simulink model "DrogueVisualNavigation_2016b"  (R2016b)
settings: Solver=ode3  StartTime=0.0  StopTime=200  FixedStep=0.02  RelTol=1e-3  EnableMultiTasking=on
libraries: visionmorphops x2, visionsinks x1, vrlib x1
settings Model: Creator=daidai  LastModifiedBy=51078
settings DataIOCC: LimitDataPoints=on  SaveFormat=Array
settings OptimizationCC: LifeSpan=inf
settings DebuggingCC: UnderspecifiedInitializationDetection=Classic  MergeDetectMultiDrivingBlocksExec=none  SolverPrmCheckMsg=warning  StateNameClashWarn=warning  SFUnexpectedBacktrackingDiag=warning  SFNoUnconditionalDefaultTransitionDiag=warning  SFExecutionAtInitializationDiag=none
settings HardwareCC: ProdBitPerPointer=32  ProdBitPerSizeT=32  ProdBitPerPtrDiffT=32  ProdLargestAtomicFloat=None  ProdIntDivRoundTo=Undefined  ProdEndianess=Unspecified  ProdWordSize=32  ProdHWDeviceType=32-bit Generic
settings ModelReferenceCC: PropagateSignalLabelsOutOfModel=off
settings GRTTargetCC: TargetLangStandard=C89/C90 (ANSI)  GeneratePreprocessorConditionals=Disable all
settings ConfigComp: CovMetricSettings=dw  CovHtmlReporting=on  CovSaveCumulativeToWorkspaceVar=on  CovSaveSingleToWorkspaceVar=on  CovExternalEMLEnable=off

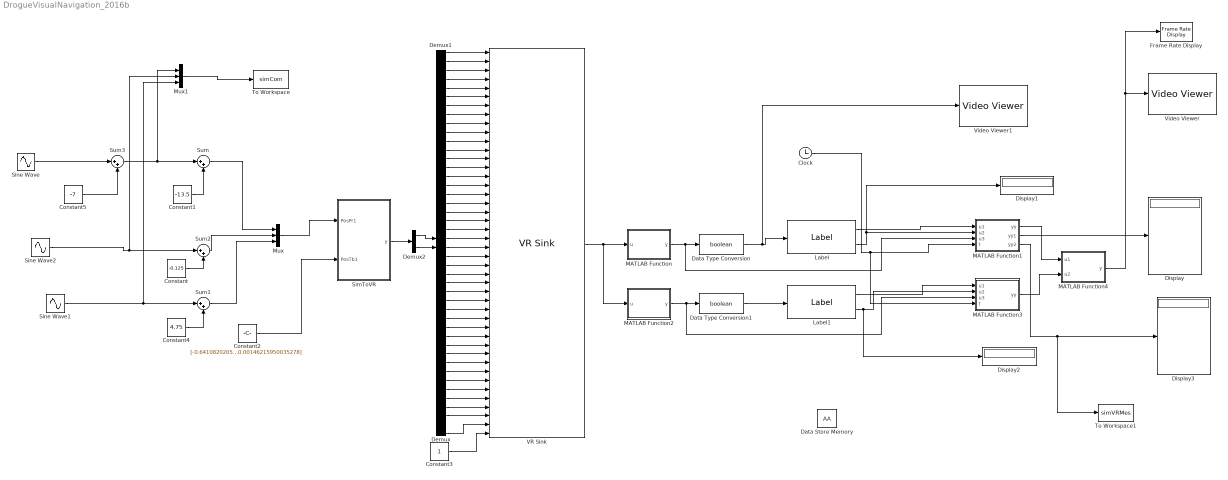
== system DrogueVisualNavigation_2016b ==
  Clock : Clock
  Constant : Constant  Value=-0.125
  Constant1 : Constant  Value=-13.5
  Constant2 : Constant  Value="[-0.641082020570737\t0.000198505356969816\t0.319485276494183\t-1.28393532402013\t-0.00160281843683540\t0.635386248124202\t-1.93123901470987\t-0.00236208899737502\t0.942069136345351\t-2.57908748233429\t-0.00371191186814384\t1.24759749734461\t-3.23222347389724\t-0.00458728864970563\t1.54165471735559\t-3.88606315497445\t-0.00765856664806413\t1.83412912153534\t-4.54441464916205\t-0.00690931267848755\t2.11631662501387\t-5.20488531429186\t-0.00757809487662455\t2.39350806000665\t-5.86949292725030\t-0.00976373475740374\t2.66062036256121\t-6.53599124911111\t-0.0104781906153184\t2.92298750019385\t-7.20684903813727\t-0.0123446852873486\t3.17399224417408\t-7.88023087161393\t-0.0124294906988970\t3.41815190003813\t-8.55684999137055\t-0.0142996532310569\t3.65318404182279\t-9.23697996759531\t-0.0159268140819394\t3.87785626126273\t-9.92032158813885\t-0.0164263298291676\t4.09256773863864\t-10.6066111675631\t-0.0169568013994899\t4.29766130307588\t-11.2962129353769\t-0.0151955417452362\t4.49131908937044\t-11.9886887378561\t-0.0139647208223945\t4.67443868542926\t-12.6842362038538\t-0.0162199773408155\t4.84551081864269\t-13.3827602154087\t-0.0151986230932412\t5.00400435326389\t0.462329282331198\t0.456745997324795\t0.442456410271379\t0.440673569146200\t0.423039498148698\t0.420617409284319\t0.404938855304994\t0.397362334614631\t0.382149787076285\t0.375020180752588\t0.358028304224740\t0.347844084701537\t0.334322083149496\t0.319050746042371\t0.304440174994498\t0.290395880255186\t0.273773209510574\t0.258523760775515\t0.241165090536005\t0.223119792668294\t-0.000309641113392978\t0.00280206863637395\t0.00117297371116799\t0.00208354420047296\t0.00134026645096743\t0.00469726065688700\t-0.00113807540912366\t0.00101258391155381\t0.00328860512426005\t0.00107195406323456\t0.00278224369822605\t0.000125939558930855\t0.00276397416973394\t0.00239242174777090\t0.000730989659109897\t0.000772955732654557\t-0.00255401872049031\t-0.00177741896870770\t0.00324240792373905\t-0.00146215950035278]"
  Constant3 : Constant
  Constant4 : Constant  Value=4.75
  Constant5 : Constant  Value=-7
  Data Store Memory : DataStoreMemory  DataStoreName=AA  InitialValue=[0 0 0]  ShowAdditionalParam=off  OutDataTypeStr=double
  Data Type Conversion : DataTypeConversion  OutDataTypeStr=boolean
  Data Type Conversion1 : DataTypeConversion  OutDataTypeStr=boolean
  Demux : Demux  Outputs=22
  Demux1 : Demux  Outputs=22
  Demux2 : Demux  Outputs=[88,66]
  Display{,1..3} (4 alike) : Display
  Frame Rate Display : visionsinks/Frame Rate Display  UpdateRate=10
  Label : visionmorphops/Label  conn=8  output=Label matrix and number of labels  outType=Automatic  lastLabel=maximum value of the output data type
  Label1 : visionmorphops/Label  conn=8  output=Label matrix and number of labels  outType=Automatic  lastLabel=maximum value of the output data type
  MATLAB Function : MATLAB Function  TreatAsAtomicUnit=on
  MATLAB Function1 : MATLAB Function  TreatAsAtomicUnit=on
  MATLAB Function2 : MATLAB Function  TreatAsAtomicUnit=on
  MATLAB Function3 : MATLAB Function  TreatAsAtomicUnit=on
  MATLAB Function4 : MATLAB Function  TreatAsAtomicUnit=on
  Mux : Mux  Inputs=3
  Mux1 : Mux  Inputs=3
  SimToVR : MATLAB Function  TreatAsAtomicUnit=on
  Sine Wave : Sin  Amplitude=7  SampleTime=0
  Sine Wave1 : Sin  Frequency=5  SampleTime=0
  Sine Wave2 : Sin  Frequency=3  SampleTime=0
  Sum{,1..3} (4 alike) : Sum  Inputs=|++
  To Workspace : ToWorkspace  VariableName=simCom  SampleTime=-1
  To Workspace1 : ToWorkspace  VariableName=simVRMes  SampleTime=-1
  VR Sink : vrlib/VR Sink  InstantiateOnLoad=on  SampleTime=-1  ViewEnable=on  RemoteChange=off  RemoteView=off  FieldsWritten=tube1.rotation.4.1.1.double#tube1.translation.3.1.1.double#tube2.rotation.4.1.1.double#tube2.translation.3.1.1.double#tube3.rotation.4.1.1.double#tube3.translation.3.1.1.double#tube4.rotation.4.1.1.double#tube4.translation.3.1.1.double#tube5.rotation.4.1.1.double#tube5.translation.3.1.1.double#tube6.rotation.4.1.1.double#tube6.translation.3.1.1.double#tube7.rotation.4.1.1.double#tube7.translation.3.1.1.double#tube8.rotation.4.1.1.double#tube8.translation.3.1.1.double#tube9.rotation.4.1.1.double#tube9.translation.3.1.1.double#tube10.rotation.4.1.1.double#tube10.translation.3.1.1.double#tube11.rotation.4.1.1.double#tube11.translation.3.1.1.double#tube12.rotation.4.1.1.double#tube12.translation.3.1.1.double#tube13.rotation.4.1.1.double#tube13.translation.3.1.1.double#tube14.rotation.4.1.1.double#tube14.translation.3.1.1.double#tube15.rotation.4.1.1.double#tube15.translation.3.1.1.double#tube16.rotation.4.1.1.double#tube16.translation.3.1.1.double#tube17.rotation.4.1.1.double#tube17.translation.3.1.1.double#tube18.rotation.4.1.1.double#tube18.translation.3.1.1.double#tube19.rotation.4.1.1.double#tube19.translation.3.1.1.double#tube20.rotation.4.1.1.double#tube20.translation.3.1.1.double#tube21.rotation.4.1.1.double#tube21.translation.3.1.1.double#ASDD.translation.3.1.1.double#ReceiverViewPoint.set_bind.1.1.1.logical  WorldFileName=AirRefuelingTubeSim.WRL  AutoView=off  VideoDimensions=[480 860]  AllowVariableSize=off  FigureProperties="{'Position', 'Name', 'Viewpoint', 'CameraBound', 'CameraDirection', 'CameraPosition', 'CameraUpVector', 'ZoomFactor', 'Antialiasing', 'Headlight', 'Lighting', 'NavPanel', 'Sound', 'StatusBar', 'Stereo3D', 'Stereo3DCameraOffset', 'Stereo3DHIT', 'ToolBar', 'Textures', 'Transparency', 'Triad', 'Wireframe', 'NavZones', 'NavMode', 'NavSpeed', 'CaptureFileFormat', 'CaptureFileName', 'Record2DCompressMethod', 'Record2DCompressQuality', 'Record2D', 'Record2DFileName', 'Record2DFPS'; [3.0000000000000000e+01   6.0000000000000000e+01   8.6000000000000000e+02   4.8000000000000000e+02], '', 'Receive1', 'on', [0.0000000000000000e+00   0.0000000000000000e+00  -1.0000000000000000e+00], [0.0000000000000000e+00   0.0000000000000000e+00   0.0000000000000000e+00], [0.0000000000000000e+00   1.0000000000000000e+00   0.0000000000000000e+00], [1.0000000000000000e+00], 'on', 'on', 'on', 'none', 'on', 'off', 'off', [1.0000000149011612e-01], [0.0000000000000000e+00], 'off', 'on', 'on', 'none', 'off', 'off', 'walk', 'normal', 'tif', '%f_anim_%n.tif', 'auto', [7.5000000000000000e+01], 'off', '***video***', [1.5000000000000000e+01]}"
  Video Viewer : VideoViewer  FigPos=[74 829 919 535]
  Video Viewer1 : VideoViewer  FigPos=[1 1110 2048 1012.8]
  wires:
  Demux2/2 -> Demux/1
  SimToVR/1(y) -> Demux2/1
  Demux2/1 -> Demux1/1
  Mux/1 -> SimToVR/1(PosPr1)
  Sum/1 -> Mux/1
  Constant2/1 -> SimToVR/2(PosTb1)
  Demux1/1 -> VR Sink/1
  Demux/1 -> VR Sink/2
  Demux1/2 -> VR Sink/3
  Demux/2 -> VR Sink/4
  Demux1/3 -> VR Sink/5
  Demux/3 -> VR Sink/6
  Demux1/4 -> VR Sink/7
  Demux/4 -> VR Sink/8
  Demux1/5 -> VR Sink/9
  Demux/5 -> VR Sink/10
  Demux1/6 -> VR Sink/11
  Demux/6 -> VR Sink/12
  Demux1/7 -> VR Sink/13
  Demux/7 -> VR Sink/14
  Demux1/8 -> VR Sink/15
  Demux/8 -> VR Sink/16
  Demux1/9 -> VR Sink/17
  Demux/9 -> VR Sink/18
  Demux1/10 -> VR Sink/19
  Demux/10 -> VR Sink/20
  Demux1/11 -> VR Sink/21
  Demux/11 -> VR Sink/22
  Demux1/12 -> VR Sink/23
  Demux/12 -> VR Sink/24
  Demux1/13 -> VR Sink/25
  Demux/13 -> VR Sink/26
  Demux1/14 -> VR Sink/27
  Demux/14 -> VR Sink/28
  Demux1/15 -> VR Sink/29
  Demux/15 -> VR Sink/30
  Demux1/16 -> VR Sink/31
  Demux/16 -> VR Sink/32
  Demux1/17 -> VR Sink/33
  Demux/17 -> VR Sink/34
  Demux1/18 -> VR Sink/35
  Demux/18 -> VR Sink/36
  Demux1/19 -> VR Sink/37
  Demux/19 -> VR Sink/38
  Demux1/20 -> VR Sink/39
  Demux/20 -> VR Sink/40
  Demux1/21 -> VR Sink/41
  Demux/21 -> VR Sink/42
  Demux/22 -> VR Sink/43
  Constant3/1 -> VR Sink/44
  VR Sink/1 -> MATLAB Function2/1(u), MATLAB Function/1(u)
  Label/1 -> MATLAB Function1/1(u1)
  MATLAB Function/1(y) -> MATLAB Function1/3(u3), Data Type Conversion/1
  Data Type Conversion/1 -> Video Viewer1/1, Label/1
  Sum1/1 -> Mux/3
  Sum2/1 -> Mux/2
  MATLAB Function2/1(y) -> MATLAB Function3/3(u3), Data Type Conversion1/1
  Data Type Conversion1/1 -> Label1/1
  Label1/1 -> MATLAB Function3/1(u1)
  Label1/2 -> Display2/1, MATLAB Function3/2(u2)
  MATLAB Function1/1(yy) -> MATLAB Function4/1(u1)
  MATLAB Function3/1(yy) -> MATLAB Function4/2(u2)
  Constant1/1 -> Sum/2
  Constant/1 -> Sum2/2
  Constant4/1 -> Sum1/2
  MATLAB Function1/2(yy1) -> Display/1
  MATLAB Function4/1(y) -> Frame Rate Display/1, Video Viewer/1
  MATLAB Function1/3(yy2) -> To Workspace1/1, Display3/1
  Clock/1 -> MATLAB Function3/4(t), MATLAB Function1/4(t)
  Sine Wave/1 -> Sum3/1
  Constant5/1 -> Sum3/2
  Label/2 -> MATLAB Function1/2(u2), Display1/1
  Sum3/1 -> Mux1/1, Sum/1
  Sine Wave2/1 -> Mux1/2, Sum2/1
  Sine Wave1/1 -> Mux1/3, Sum1/1
  Mux1/1 -> To Workspace/1

== matlab function DrogueVisualNavigation_2016b/MATLAB Function1 ==
  data: u1 input; yy output; u2 input; u3 input; yy1 output; yy2 output; t input; AA data_store_memory
function [yy,yy1,yy2] = fcn(u1,u2,u3,t)
%#codegen
L=u1;
N=u2;
Ir=u3;
t0=0.1;
global AA;
%S=zeros(N,2);
dX=zeros(10,1);
dY=zeros(10,1);
 for k=1:N
     [r,c]=find(L == k);
     dX(k)=mean(r);
     dY(k)=mean(c);     
 end
% %plot(S(:,1),S(:,2),'+')
% % dx(:,1)=S(:,1)-mean(S(:,1));
% % dy(:,1)=S(:,2)-mean(S(:,2));
% 
% dX=S(:,1);
% dY=S(:,2);

m=[dX(1:N,1) dY(1:N,1) ones(size(dX(1:N,1)))]\-(dX(1:N,1).^2+dY(1:N,1).^2);
cX=-0.5*m(1);
cY=-0.5*m(2);
cR=sqrt((m(1)^2+m(2)^2)/4-m(3));

if N==3
   AA=[cX;cY;cR]; 
end

if N<3
   cX=AA(1);
   cY=AA(2);
   cR=AA(3);
end

%yy=N;
% 
%yy = [cX,cY,cR];
%yy=[yy,N];


[mm,nn]=size(Ir);


if t>t0
    alpha=0:pi/100:2*pi;
    x=cR*cos(alpha)+cX;
    y=cR*sin(alpha)+cY;

    % if isempty(Ir)
    %     Ir=zeros(720,1280);    
    % end





    for k=1:length(alpha)

        i=floor(x(k));
        j=floor(y(k));
        if(i>=1&&j>=1&&i<=mm&&j<=nn)
            Ir(i:i,j:j)=1;        
        end

    end
end    
    
if t>t0+0.05
    i=floor(cX);
    j=floor(cY);

    if(i-3>=1&&j-3>=1&&i+4<=mm&&j+4<=nn)
        Ir(i-3:i+4,j:j+1)=1; 
        Ir(i:i+1,j-3:j+4)=1;  
    end
end

if t>t0+0.1
    i=floor(mm/2+42.57);
    j=floor(44.14+nn/2);
    if(i-3>=1&&j-3>=1&&i+4<=mm&&j+4<=nn)
        Ir(i-3:i+4,j:j+1)=1; 
        Ir(i:i+1,j-3:j+4)=1;  
    end
end

% 
% 
% 
% 
yy=Ir;

yy1=[cY-nn/2,mm/2-cX,cR];
f=196.8372/0.330;
s=196.8372/yy1(3);
xw=-s+1.928;
yw=yy1(1)*s/f-(46.94*1.862225/f);
zw=yy1(2)*s/f+(52.06*1.862225/f)-0.02;
yw=-yw;
xxw=xw*cos(5/180*pi)-zw*sin(5/180*pi);
zzw=xw*sin(5/180*pi)-zw*cos(5/180*pi);

% xw=-s+1.8925;
% 
% yw=(yy1(1)*s/2/196.9344-0.2206)/-1.4705;
% zw=(yy1(2)*s/2/196.9344+0.4953-2.9364-1.4682*xw)/1.4682;
yy2=[xxw;yw;zzw];
% yy2=[xw;yw;zw];


% function [yy,yy1,yy2] = fcn(u1,u2,u3)
% %#codegen
% L=u1;
% N=u2;
% Ir=u3;
% %S=zeros(N,2);
% dX=zeros(10,1);
% dY=zeros(10,1);
%  for k=1:N
%      [r,c]=find(L == k);
%      dX(k)=mean(r);
%      dY(k)=mean(c);     
%  end
% % %plot(S(:,1),S(:,2),'+')
% % % dx(:,1)=S(:,1)-mean(S(:,1));
% % % dy(:,1)=S(:,2)-mean(S(:,2));
% % 
% % dX=S(:,1);
% % dY=S(:,2);
% 
% m=[dX(1:N,1) dY(1:N,1) ones(size(dX(1:N,1)))]\-(dX(1:N,1).^2+dY(1:N,1).^2);
% cX=-0.5*m(1);
% cY=-0.5*m(2);
% cR=sqrt((m(1)^2+m(2)^2)/4-m(3));
% 
% 
% %yy=N;
% % 
% %yy = [cX,cY,cR];
% %yy=[yy,N];
% 
% % 
% alpha=0:pi/100:2*pi;
% x=cR*cos(alpha)+cX;
% y=cR*sin(alpha)+cY;
% 
% % if isempty(Ir)
% %     Ir=zeros(720,1280);    
% % end
% 
% [mm,nn]=size(Ir);
% for k=1:length(alpha)
% 
%     i=floor(x(k));
%     j=floor(y(k));
%     if(i>=1&&j>=1&&i<=mm&&j<=nn)
%         Ir(i:i,j:j)=1;        
%     end
%         
% end
% 
% i=floor(cX);
% j=floor(cY);
% 
% if(i-3>=1&&j-3>=1&&i+4<=mm&&j+4<=nn)
%     Ir(i-3:i+4,j:j+1)=1; 
%     Ir(i:i+1,j-3:j+4)=1;  
% end
% 
% % 
% % 
% % 
% % 
% yy=Ir;
% 
% yy1=[cY-nn/2,mm/2-cX,cR];
% 
% s=196.9344/yy1(3);
% xw=-s+1.8925;
% 
% yw=(yy1(1)*s/2/196.9344-0.2206)/-1.4705;
% zw=(yy1(2)*s/2/196.9344+0.4953-2.9364-1.4682*xw)/1.4682;
% yy2=[xw;yw;zw];
% 
%

== matlab function DrogueVisualNavigation_2016b/MATLAB Function ==
  data: u input; y output
function y = fcn(u)
%#codegen

 Ir=u(:,:,1)*2-u(:,:,2)*1-u(:,:,3)*1;

% Ir=u(:,:,1)*0.3-u(:,:,2)*0.59-u(:,:,3)*0.11

S=size(Ir);
Iin=zeros(S(1),S(2));
for i=1:S(1)
    for j=1:S(2)
       if Ir(i,j)<50
            Iin(i,j)=0;
        else
            Iin(i,j)=1;
        end
    end
end


y = Iin;

== matlab function DrogueVisualNavigation_2016b/SimToVR ==
  data: y output; PosPr1 input; PosTb1 input
function y = SimToVR(PosPr1,PosTb1)
%#codegen

%%函数名：SimToVR
%%用途  ：将软管锥套坐标输出转换为VR输入
%%输入  ：PosPr - 受油机椎管坐标， PlsTb - 软管坐标数据
%%输出  ：VrPos - 软管和受油机VR位置，VrAngle - 旋转角度输出
%%作者  ：戴训华
%%时间  ：2014/3/19

PosPr = PosPr1(1:3);
%AttitudeRecei = [PosPr1(4);-PosPr1(6);PosPr1(5)-0.115609];
AttitudeRecei=[0;-0;0-0.115609];



PosTb = PosTb1(1:60);

VrAngle = zeros(22*4,1);
VrPos = zeros(22*3,1);


for j = 1:21                        %前20为软管坐标数据，后1为软管平滑过渡处理
    if j == 1
        pX = [0, 0, 0]';            %软管起点
        pY = PosTb(3*j-2:3*j);      %软杆终点
    elseif j == 21                  %多加一段杆，做过渡
        pX = PosTb(3*j-5:3*j-3);
        pY = [PosTb(3*j-5)-0.7163*cos(8/180*pi),PosTb(3*j-4),PosTb(3*j-3)+0.7163*sin(8/180*pi)]';
    else
        pX = PosTb(3*j-5:3*j-3);
        pY = PosTb(3*j-2:3*j); 
    end
    
    pZ = (pX + pY)/2;               %中点坐标
    pZ = pZ * 8/3;                  %到VR中比例的缩放

    vAxis = [0,0,-1]';               %水平轴
    vTb = pY - pX;                  %杆的方向
    
    axis1 = null([vAxis';vTb']);%获取垂直向量
    vRot = axis1(:,1)';             %得到旋转轴
    
    if vRot(2) < 0
        vRot = -vRot;
    end
    
    VrAngle(4*j-3:4*j-1) = [vRot(1),vRot(3),vRot(2)]';
    VrAngle(4*j) = acos(vAxis'*vTb / sqrt(vAxis'*vAxis * vTb'*vTb));
    
    VrPos(3*j-2:3*j) = [pZ(1),-pZ(3),pZ(2)]';
end
%y = u;
VrAngle(85:88)=[AttitudeRecei(1);AttitudeRecei(2);AttitudeRecei(3);norm(AttitudeRecei)];
pZ = PosPr+[0 0 0]';
pZ = pZ * 8/3;
VrPos(3*22-2:3*22) = [pZ(1),-pZ(3),pZ(2)]';

y = [VrAngle;VrPos];

== matlab function DrogueVisualNavigation_2016b/MATLAB Function2 ==
  data: u input; y output
function y = fcn(u)
%#codegen

Ir=u(:,:,2)*2-u(:,:,1)*1-u(:,:,3)*1;

S=size(Ir);
Iin=zeros(S(1),S(2));
for i=1:S(1)
    for j=1:S(2)
       if Ir(i,j)<50
            Iin(i,j)=0;
        else
            Iin(i,j)=1;
       end
        
       if i/S(1)>0.8
           Iin(i,j)=0;
       end
       
    end
end


y = Iin;

== matlab function DrogueVisualNavigation_2016b/MATLAB Function3 ==
  data: u1 input; yy output; u2 input; u3 input; t input
function yy = fcn(u1,u2,u3,t)
%#codegen
L=u1;
N=u2;
Ir=u3;
t0=0.25;
%S=zeros(N,2);
dX=zeros(10,1);
dY=zeros(10,1);


 for k=1:N
     [r,c]=find(L == k);
     dX(k)=mean(r);
     dY(k)=mean(c);     
 end
% %plot(S(:,1),S(:,2),'+')
% % dx(:,1)=S(:,1)-mean(S(:,1));
% % dy(:,1)=S(:,2)-mean(S(:,2));
% 
% dX=S(:,1);
% dY=S(:,2);
[mm,nn]=size(Ir);

if N==6
   [dX_up,I]=min(dX(1:6));
   

   
   if t>t0
   aa=dX(I)-mean([dX(1:I);dX(I+1:6)]);
   bb=(max(dY(1:6))-min(dY(1:6)))/6;
   
   if abs(aa/bb)>0.2

       for i=1:6
           if(i~=I)
               for j=1:29
                   i1=floor(dX(I)+(dX(i)-dX(I))/30*j);
                   j1=floor(dY(I)+(dY(i)-dY(I))/30*j);  
                   if(i1>=1&&j1>=1&&i1<=mm&&j1<=nn)              
                       Ir(i1:i1,j1:j1)=1;         
                   end             
               end    
           end       
       end          
   
   end       
       
       

   end
   dX(I:9)=dX(I+1:10); 
   dY(I:9)=dY(I+1:10);    
end

if t>t0+0.05
    ll=4;
    if N==4
       ll=3; 
    end
    if N>6
       ll=4;
    end
    
    for i=1:ll
       for j=1:19
           i1=floor(dX(i)+(dX(i+1)-dX(i))/20*j);
           j1=floor(dY(i)+(dY(i+1)-dY(i))/20*j);  
           if(i1>=1&&j1>=1&&i1<=mm&&j1<=nn)              
               Ir(i1:i1,j1:j1)=1;         
           end             
       end          
    end     
end

% 
% 
% 
% m=[dX(1:N,1) dY(1:N,1) ones(size(dX(1:N,1)))]\-(dX(1:N,1).^2+dY(1:N,1).^2);
% cX=-0.5*m(1);
% cY=-0.5*m(2);
% cR=sqrt((m(1)^2+m(2)^2)/4-m(3));
% 
% 
% %yy=N;
% % 
% %yy = [cX,cY,cR];
% %yy=[yy,N];
% 
% % 
% alpha=0:pi/100:2*pi;
% x=cR*cos(alpha)+cX;
% y=cR*sin(alpha)+cY;
% 
% % if isempty(Ir)
% %     Ir=zeros(720,1280);    
% % end
% 
% [mm,nn]=size(Ir);
% for k=1:length(alpha)
% 
%     i=floor(x(k));
%     j=floor(y(k));
%     if(i>=1&&j>=1&&i+1<=mm&&j+1<=nn)
%         Ir(i:i+1,j:j+1)=1;        
%     end
%         
% end
% 
% i=floor(cX);
% j=floor(cY);
% 
% if(i-3>=1&&j-3>=1&&i+4<=mm&&j+4<=nn)
%     Ir(i-3:i+4,j:j+1)=1; 
%     Ir(i:i+1,j-3:j+4)=1;  
% end
% 
% % 
% 
% 
% 
yy=Ir;

== matlab function DrogueVisualNavigation_2016b/MATLAB Function4 ==
  data: u1 input; y output; u2 input
function y = fcn(u1,u2)
%#codegen

y = u1+u2;
